simulink model "test"  (R2020b)
settings: Solver=VariableStepAuto  StartTime=0.0  StopTime=10.0  RelTol=1e-3
libraries: hdlsllib x2
settings Model: Creator=Luke  LastModifiedBy=Luke

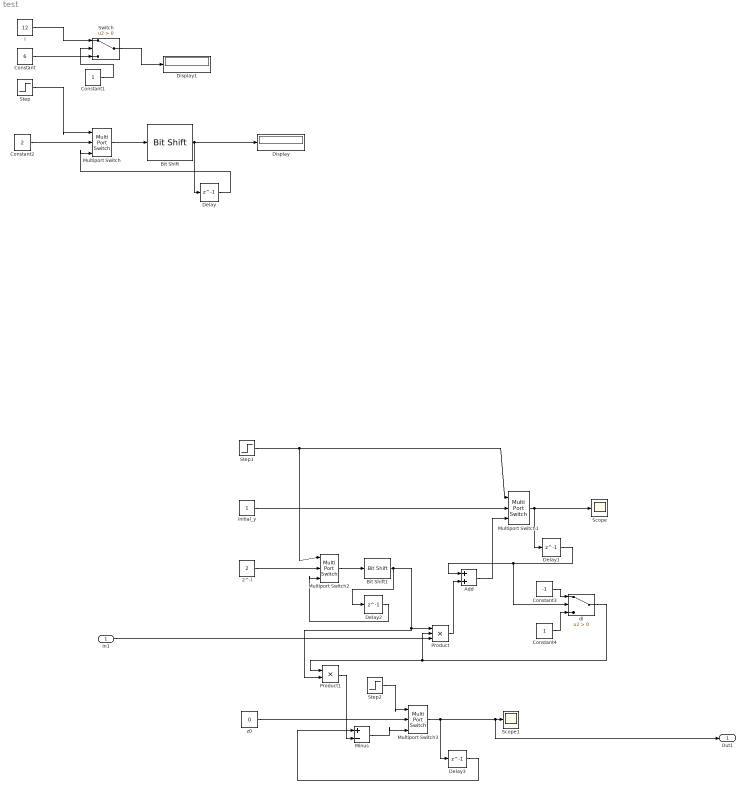
== system test ==
  In1 : Inport
  2^-i : Constant  Value=2
  Add : Sum
  Bit Shift : hdlsllib/Logic and Bit Operations/Bit Shift  mode=Shift Right Arithmetic  N=1
  Bit Shift1 : hdlsllib/Logic and Bit Operations/Bit Shift  mode=Shift Right Arithmetic  N=1
  Constant : Constant  Value=6
  Constant1 : Constant
  Constant2 : Constant  Value=2
  Constant3 : Constant  Value=-1
  Constant4 : Constant
  Delay{,1..3} (4 alike) : Delay  DelayLength=1
  Display : Display
  Display1 : Display
  Minus : Sum  Inputs=+-
  Multiport Switch{,1..3} (4 alike) : MultiPortSwitch  DataPortOrder=Zero-based contiguous  Inputs=2  zeroidx=on
  Product : Product  Inputs=3
  Product1 : Product
  Scope : Scope
  Scope1 : Scope
  Step : Step  SampleTime=0
  Step1 : Step  SampleTime=0
  Step2 : Step  SampleTime=0
  Switch : Switch  Criteria=u2 > Threshold
  di : Switch  Criteria=u2 > Threshold
  i : Constant  Value=12
  initial_y : Constant
  z0 : Constant  Value=0
  Out1 : Outport
  wires:
  Multiport Switch/1 -> Bit Shift/1
  Step/1 -> Multiport Switch/1
  Constant2/1 -> Multiport Switch/2
  Bit Shift/1 -> Delay/1, Display/1
  Delay/1 -> Multiport Switch/3
  Constant1/1 -> Switch/2
  i/1 -> Switch/1
  Constant/1 -> Switch/3
  Switch/1 -> Display1/1
  di/1 -> Product1/1, Product/2
  Delay3/1 -> Minus/1
  Multiport Switch3/1 -> Delay3/1, Out1/1, Scope1/1
  In1/1 -> Product/3
  Step2/1 -> Multiport Switch3/1
  2^-i/1 -> Multiport Switch2/2
  Constant3/1 -> di/1
  z0/1 -> Multiport Switch3/2
  Bit Shift1/1 -> Delay2/1, Product1/2, Product/1
  Delay2/1 -> Multiport Switch2/3
  Step1/1 -> Multiport Switch2/1, Multiport Switch1/1
  Delay1/1 -> di/2, Add/1
  Minus/1 -> Multiport Switch3/3
  initial_y/1 -> Multiport Switch1/2
  Constant4/1 -> di/3
  Product/1 -> Add/2
  Add/1 -> Multiport Switch1/3
  Multiport Switch2/1 -> Bit Shift1/1
  Multiport Switch1/1 -> Delay1/1, Scope/1
  Product1/1 -> Minus/2
